simulink model "Steps_count"  (R2021b)
settings: Solver=VariableStepAuto  StartTime=0.0  StopTime=10.0  RelTol=1e-3
undefined symbols (not defined in the file or in its folder): fdesignblkfcn, gcbh, magnitude
libraries: dspstat3 x3, androidsensorlib x1, androiduilib x1
settings Model: Creator=cristinaquagliozzi  LastModifiedBy=cristinaquagliozzi

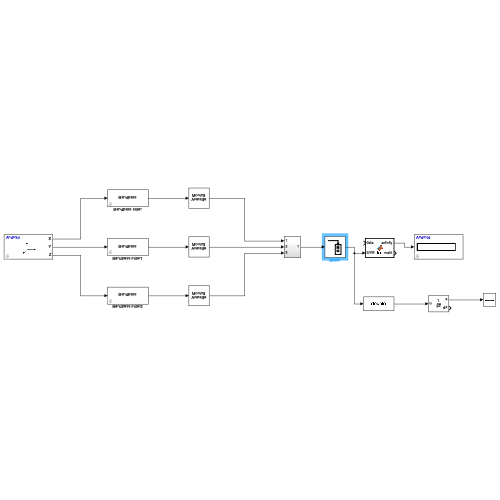
[thumbnail: Simulink's stored preview of the top-level diagram]
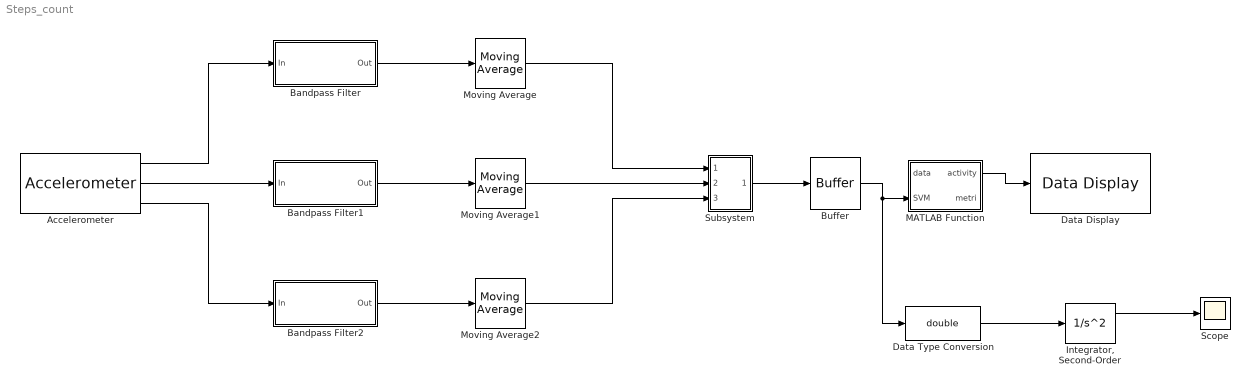
== system Steps_count ==
  Accelerometer : androidsensorlib/Accelerometer  OutputVector=off  SampleTime=0.05  BlockPlatform=Android
      settings: SourceProductBaseCode=ANDROID
  Bandpass Filter : Subsystem  DialogController=fdesignblkfcn  InitFcn=fdesignblkfcn(gcbh, {'InitFcn'});  mask(Bandpass Filter){}
      mask help: Design a bandpass filter
      settings: CopyFcn=fdesignblkfcn(gcbh, {'CopyFcn'});
      mask Help: helpview(mapfilelocation('dsp'), 'dspbandpassfilter');
      mask Display: disp('Bandpass');
  Bandpass Filter1 : Subsystem  DialogController=fdesignblkfcn  InitFcn=fdesignblkfcn(gcbh, {'InitFcn'});  mask(Bandpass Filter){}
      mask help: Design a bandpass filter
      settings: CopyFcn=fdesignblkfcn(gcbh, {'CopyFcn'});
      mask Help: helpview(mapfilelocation('dsp'), 'dspbandpassfilter');
      mask Display: disp('Bandpass');
  Bandpass Filter2 : Subsystem  DialogController=fdesignblkfcn  InitFcn=fdesignblkfcn(gcbh, {'InitFcn'});  mask(Bandpass Filter){}
      mask help: Design a bandpass filter
      settings: CopyFcn=fdesignblkfcn(gcbh, {'CopyFcn'});
      mask Help: helpview(mapfilelocation('dsp'), 'dspbandpassfilter');
      mask Display: disp('Bandpass');
  Buffer : Buffer  N=500  OutputFrames=off
  Data Display : androiduilib/Data Display  Format=Float  Precision=6  SimulateUsing=Code generation  blockPlatform=Android
      settings: SourceProductBaseCode=ANDROID
  Data Type Conversion : DataTypeConversion  OutDataTypeStr=double
  "Integrator, Second-Order" : SecondOrderIntegrator
  MATLAB Function : MATLAB Function  TreatAsAtomicUnit=on
  Moving Average : dspstat3/Moving Average  Method=Sliding window  ForgettingFactorPort=off  SpecifyWindowLength=on  WindowLength=4  ForgettingFactor=0.9  SimulateUsing=Code generation
  Moving Average1 : dspstat3/Moving Average  Method=Sliding window  ForgettingFactorPort=off  SpecifyWindowLength=on  WindowLength=4  ForgettingFactor=0.9  SimulateUsing=Code generation
  Moving Average2 : dspstat3/Moving Average  Method=Sliding window  ForgettingFactorPort=off  SpecifyWindowLength=on  WindowLength=4  ForgettingFactor=0.9  SimulateUsing=Code generation
  Scope : Scope
  Subsystem : Subsystem
  wires:
  Accelerometer/1 -> Bandpass Filter/1(In)
  Accelerometer/2 -> Bandpass Filter1/1(In)
  Accelerometer/3 -> Bandpass Filter2/1(In)
  Bandpass Filter2/1(Out) -> Moving Average2/1
  Bandpass Filter1/1(Out) -> Moving Average1/1
  Bandpass Filter/1(Out) -> Moving Average/1
  Moving Average/1 -> Subsystem/1(In1)
  Moving Average1/1 -> Subsystem/2(In2)
  Moving Average2/1 -> Subsystem/3(In3)
  Subsystem/1(Out1) -> Buffer/1
  Buffer/1 -> Data Type Conversion/1, MATLAB Function/2(SVM)
  MATLAB Function/1(activity) -> Data Display/1
  Data Type Conversion/1 -> "Integrator, Second-Order"/1
  "Integrator, Second-Order"/1 -> Scope/1

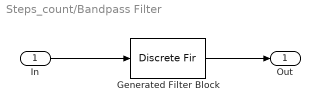
== system Steps_count/Bandpass Filter ==
  In : Inport
  Generated Filter Block : DiscreteFir  Tag=BlockMethodSubSystem  Coefficients=[0.0356981661093621061 0.241086532539355275 0.446533045298186826 0.241086532539355275 0.0356981661093621061]  InputProcessing=Columns as channels (frame based)
  Out : Outport  VectorParamsAs1DForOutWhenUnconnected=off
  wires:
  In/1 -> Generated Filter Block/1
  Generated Filter Block/1 -> Out/1

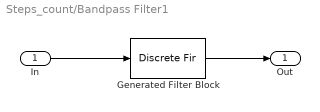
== system Steps_count/Bandpass Filter1 ==
  In : Inport
  Generated Filter Block : DiscreteFir  Tag=BlockMethodSubSystem  Coefficients=[0.0356981661093621061 0.241086532539355275 0.446533045298186826 0.241086532539355275 0.0356981661093621061]  InputProcessing=Columns as channels (frame based)
  Out : Outport  VectorParamsAs1DForOutWhenUnconnected=off
  wires:
  In/1 -> Generated Filter Block/1
  Generated Filter Block/1 -> Out/1

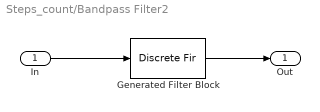
== system Steps_count/Bandpass Filter2 ==
  In : Inport
  Generated Filter Block : DiscreteFir  Tag=BlockMethodSubSystem  Coefficients=[0.0356981661093621061 0.241086532539355275 0.446533045298186826 0.241086532539355275 0.0356981661093621061]  InputProcessing=Columns as channels (frame based)
  Out : Outport  VectorParamsAs1DForOutWhenUnconnected=off
  wires:
  In/1 -> Generated Filter Block/1
  Generated Filter Block/1 -> Out/1

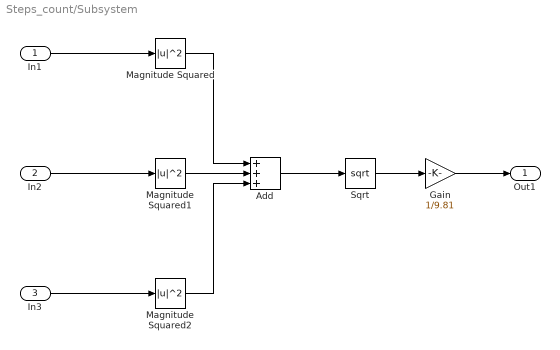
== system Steps_count/Subsystem ==
  In1 : Inport
  In2 : Inport  Port=2
  In3 : Inport  Port=3
  Add : Sum  Inputs=+++
  Gain : Gain  Gain=1/9.81
  Magnitude Squared : Math  Operator=magnitude^2  SaturateOnIntegerOverflow=on
  Magnitude Squared1 : Math  Operator=magnitude^2  SaturateOnIntegerOverflow=on
  Magnitude Squared2 : Math  Operator=magnitude^2  SaturateOnIntegerOverflow=on
  Sqrt : Sqrt  SaturateOnIntegerOverflow=on
  Out1 : Outport
  wires:
  In3/1 -> Magnitude Squared2/1
  Gain/1 -> Out1/1
  In1/1 -> Magnitude Squared/1
  Magnitude Squared1/1 -> Add/2
  Sqrt/1 -> Gain/1
  Magnitude Squared2/1 -> Add/3
  Add/1 -> Sqrt/1
  In2/1 -> Magnitude Squared1/1
  Magnitude Squared/1 -> Add/1

== matlab function Steps_count/MATLAB Function ==
  data: data input; SVM input; activity output; metri output
function [activity, metri] = fcn(data, SVM)

threshold_1=1.02;
threshold_2=2.5;
activity= 1;

%lista = 0 ; inizializzatra 

if max(SVM)<=threshold_1
    activity=1; %riposo
elseif max(SVM) > threshold_2 && max(SVM)<= threshold_2
    activity=2; %camminata 
    lista = lista + 1;
elseif max(SVM)>threshold_2
    activity=3; %corsa 

metri = lista * 0.1*0.7;
end
